simulink subsystem "turn_off_system"  (R2022b)
settings: Solver=VariableStepAuto  StartTime=0.0  StopTime=inf  RelTol=1e-3
settings Model: DefaultTestHarness=turn_off_system_Harness1  Creator=pppc  LastModifiedBy=pppc

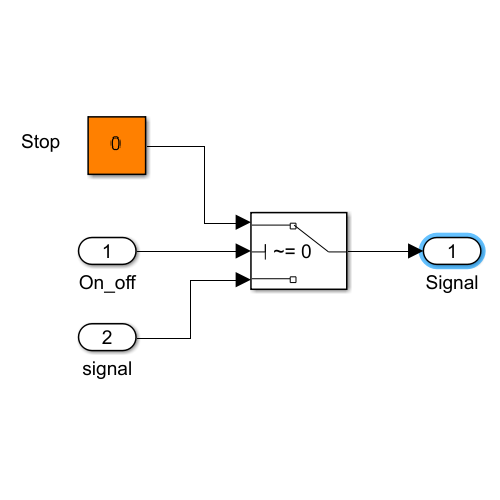
[thumbnail: Simulink's stored preview of the top-level diagram]
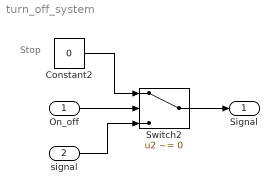
== system turn_off_system ==
  note: Stop
  On_off : Inport
  signal : Inport  Port=2
  Constant2 : Constant  Value=0
  Switch2 : Switch  Criteria=u2 ~= 0  SaturateOnIntegerOverflow=off  InputSameDT=off
  Signal : Outport
  wires:
  Constant2/1 -> Switch2/1
  signal/1 -> Switch2/3
  On_off/1 -> Switch2/2
  Switch2/1 -> Signal/1
